simulink model "GesamtmodellII"  (Simulink 8.3)
settings: Solver=ode45  StartTime=0.0  StopTime=10  RelTol=1e-3
values from neighbouring files (symbols this model uses):
  JR = 0.00000198    (= 1.98e-06)    [EingabparameterI.m]
  k1 = 3.4/(1000/60)    (= 0.204)    [EingabparameterI.m]
  k2 = 0.0325    [EingabparameterI.m]
  KRI1 = 0.03    [EingabparameterI.m]
  KRI2 = 0.015    [EingabparameterI.m]
  ML = 5e-4    (= 0.0005)    [EingabparameterI.m]
  MR = k2*I0    (= 0.0008125)    [EingabparameterI.m]
  RA = 5.8    [EingabparameterI.m]
  tel = LA/RA    (= 0.000129310344828)    [EingabparameterI.m]
  TN1 = 3.5    [EingabparameterI.m]
  TN2 = 0.25    [EingabparameterI.m]
  TRI1 = 0.05    [EingabparameterI.m]
  TRI2 = 0.005    [EingabparameterI.m]
undefined symbols (not defined in the file or in its folder): sigbuilder_block
CloseFcn:
  | rtwprivate ssgencode ModelCloseRequest GesamtmodellII
settings Model: Creator=mama  LastModifiedBy=hp
settings OptimizationCC: ExpressionDepthLimit=2147483647  InitFltsAndDblsToZero=on
settings DebuggingCC: FcnCallInpInsideContextMsg=UseLocalSettings  StrictBusMsg=Warning
settings RTWCC: ProcessScript=grt_make_rtw_hook
settings GRTTargetCC: CombineOutputUpdateFcns=on  GRTInterface=off

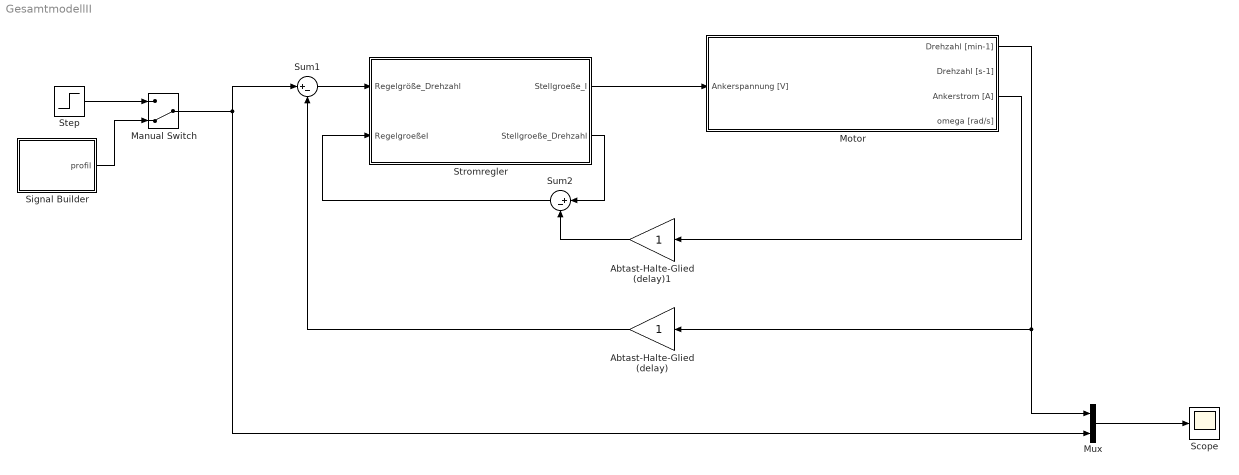
== system GesamtmodellII ==
  Abtast-Halte-Glied (delay) : Gain  SampleTime=TRI1
  Abtast-Halte-Glied (delay)1 : Gain  SampleTime=TRI2
  Manual Switch : ManualSwitch  CurrentSetting=0
  Motor : Subsystem
  Mux : Mux  Inputs=2
  Scope : Scope
      settings: YMin=1250  YMax=1300  MaxDataPoints=5000000
  Signal Builder : Subsystem  Tag=STV Subsys  LoadFcn=sigbuilder_block('load');  StartFcn=sigbuilder_block('start');  StopFcn=sigbuilder_block('stop');  ClipboardFcn=sigbuilder_block('clipboard');  mask(Sigbuilder block){}
      mask help: Sigbuilder GUI
      mask init:
      | if ~strcmp(get_param(bdroot(gcbh),'SimulationStatus'),'stopped') tuvar = sigbuilder_block('maskInit'); end
      settings: CopyFcn=sigbuilder_block('copy');  DeleteFcn=sigbuilder_block('delete');  ModelCloseFcn=sigbuilder_block('modelClose');  PreSaveFcn=sigbuilder_block('preSave');  PauseFcn=sigbuilder_block('pause')  ContinueFcn=sigbuilder_block('continue')  NameChangeFcn=sigbuilder_block('namechange');  OpenFcn=sigbuilder_block('open',[220.5 63 550.5 399.75 ]);  CloseFcn=sigbuilder_block('close');
      mask Display: plot(0,0,100,100,[10,10,40,40,10],[80,20,20,80,80],[40,10],[50,50], [40,27,10],[65,72,56],[40,25,25,10],[28,28,43,43]);
  Step : Step  Time=0  After=1300  SampleTime=0
  Stromregler : Subsystem
  Sum1 : Sum  Inputs=|+-  SampleTime=TRI1
  Sum2 : Sum  Inputs=|+-  SampleTime=TRI2
  wires:
  Motor/1(Drehzahl [min-1]) -> Mux/1, Abtast-Halte-Glied (delay)/1
  Stromregler/1(Stellgroeße_I) -> Motor/1(Ankerspannung [V])
  Step/1 -> Manual Switch/1
  Signal Builder/1(profil) -> Manual Switch/2
  Mux/1 -> Scope/1
  Manual Switch/1 -> Mux/2, Sum1/1
  Motor/3(Ankerstrom [A]) -> Abtast-Halte-Glied (delay)1/1
  Abtast-Halte-Glied (delay)/1 -> Sum1/2
  Sum1/1 -> Stromregler/1(Regelgröße_Drehzahl)
  Stromregler/2(Stellgroeße_Drehzahl) -> Sum2/1
  Abtast-Halte-Glied (delay)1/1 -> Sum2/2
  Sum2/1 -> Stromregler/2(RegelgroeßeI)

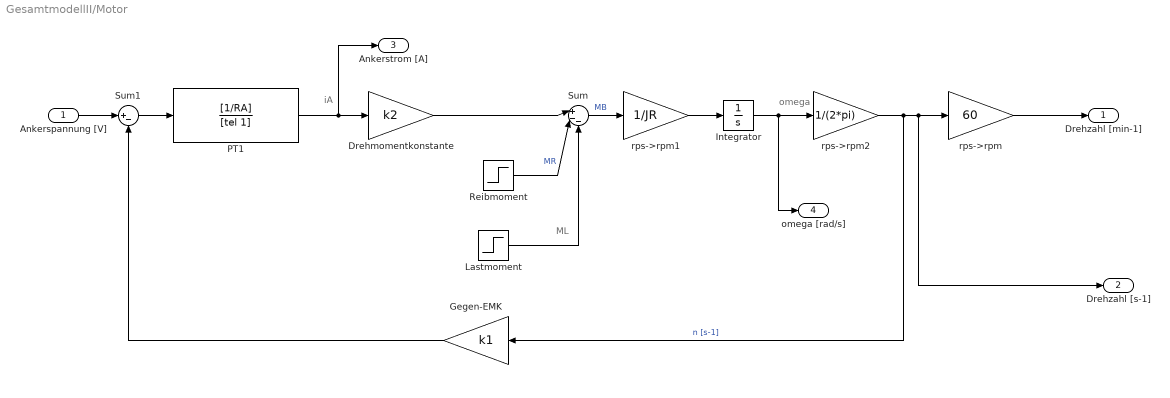
== system GesamtmodellII/Motor ==
  note: iA
  note: ML
  note: omega
  Ankerspannung [V] : Inport
  Drehmomentkonstante : Gain  Gain=k2
  Gegen-EMK : Gain  Gain=k1
  Integrator : Integrator
  Lastmoment : Step  Time=6  After=ML  SampleTime=0
  PT1 : TransferFcn  Numerator=[1/RA]  Denominator=[tel 1]
  Reibmoment : Step  Time=0  After=MR  SampleTime=0
  Sum : Sum  Inputs=|+--
  Sum1 : Sum  Inputs=|+-
  rps->rpm : Gain  Gain=60
  rps->rpm1 : Gain  Gain=1/JR
  rps->rpm2 : Gain  Gain=1/(2*pi)
  Drehzahl [min-1] : Outport
  Drehzahl [s-1] : Outport  Port=2
  Ankerstrom [A] : Outport  Port=3
  omega [rad/s] : Outport  Port=4
  wires:
  PT1/1 -> Drehmomentkonstante/1, Ankerstrom [A]/1
  Drehmomentkonstante/1 -> Sum/1
  Sum/1 -> rps->rpm1/1  "MB"
  Sum1/1 -> PT1/1
  Ankerspannung [V]/1 -> Sum1/1
  Gegen-EMK/1 -> Sum1/2
  rps->rpm/1 -> Drehzahl [min-1]/1
  Reibmoment/1 -> Sum/2  "MR"
  rps->rpm1/1 -> Integrator/1
  Integrator/1 -> rps->rpm2/1, omega [rad/s]/1
  rps->rpm2/1 -> Gegen-EMK/1, rps->rpm/1, Drehzahl [s-1]/1  "n [s-1]"
  Lastmoment/1 -> Sum/3

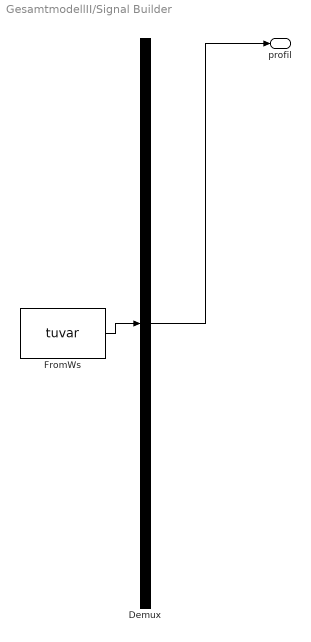
== system GesamtmodellII/Signal Builder ==
  Demux : Demux  Tag=STV Demux  Outputs=1
  FromWs : FromWorkspace  Tag=STV FromWs  VariableName=tuvar  SampleTime=0  SigBuilderData=DataTag0  VnvData=DataTag1
      SigBuilderData=|
      | common.afterFinalStr = 'Extrapolate'
      | common.sampleTime = 0
      | dataSet.timeRange = [0 10]
      | dataSet.name = 'Group 1'
      | sbobj.Name = 'Signal Builder'
      | sbobj.Groups.Name = 'Group 1'
      | sbobj.Groups.Signals.Name = 'profil'
      | sbobj.Groups.Signals.XData = [0 1 1 3 5.02 8 8.92 10]
      | sbobj.Groups.Signals.YData = [0 1940 1979.6 2000 -1980 -2000 0 -20.2]
  profil : Outport  Tag=STV Outport
  wires:
  Demux/1 -> profil/1
  FromWs/1 -> Demux/1

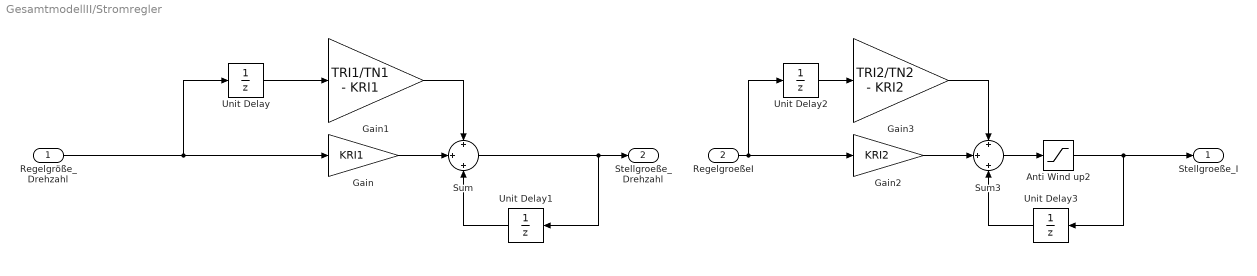
== system GesamtmodellII/Stromregler ==
  Regelgröße_Drehzahl : Inport
  RegelgroeßeI : Inport  Port=2
  Anti Wind up2 : Saturate  UpperLimit=9  LowerLimit=-9  SampleTime=TRI2
  Gain : Gain  Gain=KRI1  SampleTime=TRI1
  Gain1 : Gain  Gain=TRI1/TN1 - KRI1  SampleTime=TRI1
  Gain2 : Gain  Gain=KRI2  SampleTime=TRI2
  Gain3 : Gain  Gain=TRI2/TN2 - KRI2  SampleTime=TRI2
  Sum : Sum  Inputs=+|+|+  SampleTime=TRI1
  Sum3 : Sum  Inputs=+|+|+  SampleTime=TRI2
  Unit Delay : UnitDelay  SampleTime=TRI1
  Unit Delay1 : UnitDelay  SampleTime=TRI1
  Unit Delay2 : UnitDelay  SampleTime=TRI2
  Unit Delay3 : UnitDelay  SampleTime=TRI2
  Stellgroeße_I : Outport
  Stellgroeße_Drehzahl : Outport  Port=2
  wires:
  Sum/1 -> Unit Delay1/1, Stellgroeße_Drehzahl/1
  Gain/1 -> Sum/2
  Unit Delay1/1 -> Sum/3
  Unit Delay/1 -> Gain1/1
  Gain1/1 -> Sum/1
  Sum3/1 -> Anti Wind up2/1
  Gain2/1 -> Sum3/2
  Unit Delay3/1 -> Sum3/3
  Unit Delay2/1 -> Gain3/1
  Gain3/1 -> Sum3/1
  Anti Wind up2/1 -> Unit Delay3/1, Stellgroeße_I/1
  RegelgroeßeI/1 -> Gain2/1, Unit Delay2/1
  Regelgröße_Drehzahl/1 -> Gain/1, Unit Delay/1
